simulink model "master_model"  (R2020a)
settings: Solver=FixedStepDiscrete  StartTime=0.0  StopTime=1000.0  RelTol=1e-3  EnableMultiTasking=on
settings Model: SILPILModeSetting=veronly  ExtModeTrigDuration=2  Creator=davood  LastModifiedBy=davood
settings OptimizationCC: EnhancedBackFolding=on  PassReuseOutputArgsAs=Individual arguments  ZeroExternalMemoryAtStartup=off  ZeroInternalMemoryAtStartup=off  MaxStackSize=64  OptimizeBlockOrder=speed  DifferentSizesBufferReuse=on  OptimizationCustomize=off  EfficientTunableParamExpr=on
settings DebuggingCC: ParameterTunabilityLossMsg=error
settings HardwareCC: ProdBitPerInt=16  ProdBitPerPointer=16  ProdBitPerSizeT=16  ProdBitPerPtrDiffT=16  ProdLargestAtomicFloat=None  ProdWordSize=8  ProdHWDeviceType=Atmel->AVR
settings SFSimCC: MATLABDynamicMemAlloc=off
settings RTWCC: SystemTargetFile=ert.tlc  HardwareBoard=Arduino Uno  TLCOptions=-aInlineSetEventsForThisBaseRateFcn=TLC_FALSE -aSuppressMultiTaskScheduler=TLC_FALSE -aRateBasedStepFcn=1  TemplateMakefile=ert_default_tmf  GenerateReport=on  Toolchain=Arduino AVR  BuildConfiguration=Faster Runs  LaunchReport=on
settings CodeAppCC: ForceParamTrailComments=on  IgnoreCustomStorageClasses=off  OperatorAnnotations=on  SimulinkDataObjDesc=on  SFDataObjDesc=on  InsertBlockDesc=on
settings ERTTargetCC: SupportContinuousTime=on  SupportVariableSizeSignals=on  ExtModeStaticAllocSize=250

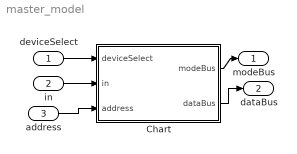
== system master_model ==
  deviceSelect : Inport
  in : Inport  Port=2
  address : Inport  Port=3
  Chart : Stateflow chart  TreatAsAtomicUnit=on
  modeBus : Outport
  dataBus : Outport  Port=2
  wires:
  Chart/2(dataBus) -> dataBus/1
  Chart/1(modeBus) -> modeBus/1
  deviceSelect/1 -> Chart/1(deviceSelect)
  in/1 -> Chart/2(in)
  address/1 -> Chart/3(address)

== stateflow chart master_model/Chart ==
  state init
  state initSend
  state addressSend
  state sendMsg
  state getReport
  (default) -> init
  init -> initSend : [deviceSelect==1 || deviceSelect==2]{dataBus=1}
  initSend -> addressSend : {dataBus=address}
  sendMsg -> init [order 2] : [deviceSelect==1 || deviceSelect==2]{dataBus=0}
  addressSend -> getReport : {modeBus=1}
  getReport -> sendMsg : {modeBus=0; dataBus=in}
  sendMsg -> getReport [order 1] : [deviceSelect ~=1 && deviceSelect~=2]{modeBus=1}
  data: modeBus output uint8; dataBus output uint8; deviceSelect input uint8; in input uint8; address input uint8
